simulink model "example_IceStorage"  (R2018b)
settings: Solver=ode45  StartTime=0.0  StopTime=5*24*3600  MaxStep=600  RelTol=1e-4  AbsTol=1e-6  EnableMultiTasking=on
undefined symbols (not defined in the file): path_carnot
libraries: carnot x11
settings Model: Creator=drhf  LastModifiedBy=drhf
settings SolverCC: AutoScaleAbsTol=off  ZeroCrossAlgorithm=Adaptive
settings DataIOCC: LimitDataPoints=on  SaveFormat=Array
settings OptimizationCC: ExpressionDepthLimit=2147483647  LifeSpan=inf
settings DebuggingCC: UnderspecifiedInitializationDetection=Classic  MergeDetectMultiDrivingBlocksExec=none  SolverPrmCheckMsg=warning  StateNameClashWarn=warning  SFUnexpectedBacktrackingDiag=warning  SFNoUnconditionalDefaultTransitionDiag=warning  SFExecutionAtInitializationDiag=none
settings HardwareCC: ProdBitPerPointer=32  ProdBitPerSizeT=32  ProdBitPerPtrDiffT=32  ProdLargestAtomicFloat=None  ProdIntDivRoundTo=Undefined  ProdEndianess=Unspecified  ProdWordSize=32  ProdHWDeviceType=32-bit Generic
settings ModelReferenceCC: PropagateSignalLabelsOutOfModel=off
settings SFSimCC: SimUseLocalCustomCode=off
settings RTWCC: RTWUseLocalCustomCode=off
settings CodeAppCC: StateflowObjectComments=on
settings GRTTargetCC: TargetLangStandard=C89/C90 (ANSI)  GeneratePreprocessorConditionals=Disable all  CombineOutputUpdateFcns=off  GRTInterface=on
settings ConfigComp: CovMetricSettings=dw  CovHtmlReporting=on  CovSaveCumulativeToWorkspaceVar=on  CovSaveSingleToWorkspaceVar=on  CovExternalEMLEnable=off

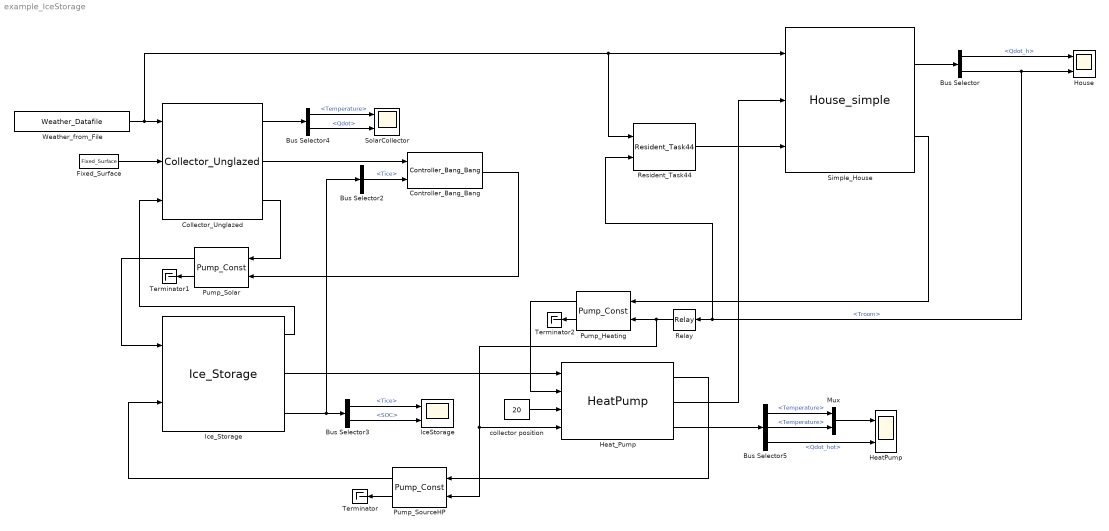
== system example_IceStorage ==
  Bus Selector : BusSelector  OutputSignals=Qdot.Qdot_h,Troom
  Bus Selector2 : BusSelector  OutputSignals=T.Tice
  Bus Selector3 : BusSelector  OutputSignals=T.Tice,SOC
  Bus Selector4 : BusSelector  OutputSignals=THBout.Temperature,Qdot
  Bus Selector5 : BusSelector  OutputSignals=THBin_cold.Temperature,THBout_hot.Temperature,Qdot_hot
  Collector_Unglazed : carnot/Source/Solar_Thermal/Collector_Unglazed  tini=20  Ncollector=1  PathName=fullfile(path_carnot('libsl'), 'Source', 'Solar_Thermal', 'Collector_Unglazed', 'parameter_set')  FileName='DefaultCollectorUnglazed.mat'  userPath=off  userParam=off  acol=2.5  len=2  nodes=10  fta=0.9  eps=0.9  u0l=40  u0c=1  u0g=40  u1l=8  u1c=1  u1g=8  u1e=0.01  hi=200  capa=5000  capf=4000  SensorTimeConstant=10  dplin=5504.4  dpqua=6222.096
      settings: SourceProductName=Carnot
  Controller_Bang_Bang : carnot/Control/Controller_Bang_Bang  deltaTon=5  deltaToff=1  Tmax=95
      settings: SourceProductName=Carnot
  Fixed_Surface : carnot/Weather/Fixed_Surface  colangle=30  colazi=0  colrot=0
      settings: SourceProductName=Carnot
  HeatPump : Scope  NumInputPorts=2
  Heat_Pump : carnot/Source/Heat_Pump/HeatPump  PathName=fullfile(path_carnot('libsl'), 'Source','Heat_Pump','HeatPump','parameter_set')  FileName='DefaultHeatPump.mat'  userPath=off  userParam=off  K=[299.999998982327 -59.9999988176087 12249.9999711932 -6.66666603880034 60.0000010482174 -5.13158332307255e-05 306.666667839537 -115.000000230844 12225.0000010917]  caph=32000  capc=32000  UA=6  relQdotMin=1  linc=10  quac=100  linh=10  quah=100
      settings: SourceProductName=Carnot
  House : Scope  NumInputPorts=2
  IceStorage : Scope  NumInputPorts=2
  Ice_Storage : carnot/Storage/Thermal/Ice_Storage  vol=10  h=2.3  z=3.32-0.12  Lhx_sol=195  Ulen_sol="1500/28/9.5            % 1.5 kW at dT = 9.5 K with a 28 m tube of outer diameter 32 mm"  mpc_sol=1*3500  Lhx_hp=7*50  Ulen_hp="1500/28/9.5            % 1.5 kW at dT = 9.5 K with a 28 m tube of outer diameter 32 mm"  mpc_hp=1*3500  dearth=0.5  cond_ground=2  cp_ground=800  rho_ground=2500  Tmeanoutside=11  deltathetae=9.3  tshift=319  f_ice=0  t_ini=15
      settings: SourceProductName=Carnot
  Mux : Mux  Inputs=2
  Pump_Heating : carnot/Hydraulics/Pump_Const  mdotmax=1200/3600  dia=0.0157  p0=3e5  fluid_id=Water  mix=0  mix2=0  mix3=0  UA=3  mcp=4000  Tini=20  e0=10  e1=10  e2=-1
      settings: SourceProductName=Carnot
  Pump_Solar : carnot/Hydraulics/Pump_Const  mdotmax=1200/3600  dia=0.0157  p0=3e5  fluid_id=Water  mix=0  mix2=0  mix3=0  UA=3  mcp=4000  Tini=20  e0=10  e1=10  e2=-1
      settings: SourceProductName=Carnot
  Pump_SourceHP : carnot/Hydraulics/Pump_Const  mdotmax=2000/3600  dia=0.0157  p0=3e5  fluid_id=Water  mix=0  mix2=0  mix3=0  UA=3  mcp=4000  Tini=20  e0=10  e1=10  e2=-1
      settings: SourceProductName=Carnot
  Relay : Relay  OnSwitchValue=20.2  OffSwitchValue=19.8  OnOutputValue=0  OffOutputValue=1
  Resident_Task44 : carnot/Load/Houses/Resident_Task44  period=24*3600  rep_seq_te=[0 1 6 7 8 9 11 12 13 18 19 20 22 23]*3600  rep_seq_de=[1 5 1 1 1 2 1 1 4 2 1 2 1 1]*3600  rep_seq_ye=[105 55 392.5 457.5 420 55 250 55 120 170 615 420 442.5 355]  rep_seq_to=[0 6 7 8 9 11 12 13 14 15 17 18 20 21 22]*3600  rep_seq_do=[6 1 1 1 2 1 1 1 1 2 1 2 1 1 2]*3600  rep_seq_yo=[4 2 3 2 0 1 3 2 1 0 1 2 4 3 4]*60  Topen=24  Tclose=23  TrAboveTa=2  TaTooCold=12  timeFIR=24  TaIni=12  starttime=8  stoptime=22  TroomShadeOn=23.8  TroomShadeOff=22.8  SolarShadeOn=300  SolarShadeOff=200  max_shade=1  CalcAirComp=off  mdotCO2=0  mdotH2O=0  mdotVOC=0
      settings: SourceProductName=Carnot
  Simple_House : carnot/Load/Houses/House_simple  tini=20  dtroom=inf  Tmeaninside=23.8  deltathetai=3.8  Tmeanoutside=11  deltathetae=9.3  tshift=319*3600  PathName=fullfile(path_carnot('libsl'), 'Load', 'Houses', 'House_simple', 'parameter_set')  FileName='<user defined>'  userPath=off  userParam=on  Ahabit=140  Hroom=2.5  slabwidth=10  slablength=7  dwall=0.4  UAwall=100  capa=500000  utot=0.183  gammat=0  cond_ground=2  cp_ground=800  rho_ground=2500  Awindow=[12 4 3 4]  AziWin=[0 90 -180 -90]  Uwindow=[2 2 2 2]  Gwindow=[0.5 0.5 0.5 0.5]  alpha=10  H=1.2  W=1  Nwin=4  Ventilationrate=0.4  Heatrecovery=0  pnom=10000  dtnom=12.5  expo=0.8  mcap=500*4812  lin=100  qua=100
      settings: SourceProductName=Carnot
  SolarCollector : Scope  NumInputPorts=2
  Terminator : Terminator
  Terminator1 : Terminator
  Terminator2 : Terminator
  Weather_from_File : carnot/Weather/Weather_Datafile  PathName=path_carnot('data')  FileName='DE_TRY2010_04_averageYear.mat'  UserParam=off  VariableName=DE_TRY2010_04_averageYear  SampleTime=3600
      settings: SourceProductName=Carnot
  collector position : Constant  Value=20
  wires:
  Bus Selector/2 -> House/2, Resident_Task44/2, Relay/1  "<Troom>"
  Heat_Pump/2 -> Simple_House/2
  Simple_House/1 -> Bus Selector/1
  Simple_House/2 -> Pump_Heating/1
  Pump_Heating/1 -> Heat_Pump/2
  Relay/1 -> Pump_Heating/2, Pump_SourceHP/2, Heat_Pump/4
  Ice_Storage/2 -> Heat_Pump/1
  Collector_Unglazed/3 -> Pump_Solar/1
  Pump_Solar/1 -> Ice_Storage/1
  Ice_Storage/1 -> Collector_Unglazed/3
  Heat_Pump/1 -> Pump_SourceHP/1
  Ice_Storage/3 -> Bus Selector3/1, Bus Selector2/1
  Controller_Bang_Bang/1 -> Pump_Solar/2
  Collector_Unglazed/2 -> Controller_Bang_Bang/1
  Bus Selector2/1 -> Controller_Bang_Bang/2  "<Tice>"
  Pump_SourceHP/1 -> Ice_Storage/2
  Fixed_Surface/1 -> Collector_Unglazed/2
  collector position/1 -> Heat_Pump/3
  Bus Selector3/1 -> IceStorage/1  "<Tice>"
  Bus Selector3/2 -> IceStorage/2  "<SOC>"
  Bus Selector4/1 -> SolarCollector/1  "<Temperature>"
  Bus Selector4/2 -> SolarCollector/2  "<Qdot>"
  Heat_Pump/3 -> Bus Selector5/1
  Bus Selector5/3 -> HeatPump/2  "<Qdot_hot>"
  Bus Selector5/1 -> Mux/1  "<Temperature>"
  Bus Selector5/2 -> Mux/2  "<Temperature>"
  Mux/1 -> HeatPump/1
  Pump_SourceHP/2 -> Terminator/1
  Pump_Solar/2 -> Terminator1/1
  Pump_Heating/2 -> Terminator2/1
  Bus Selector/1 -> House/1  "<Qdot_h>"
  Collector_Unglazed/1 -> Bus Selector4/1
  Resident_Task44/1 -> Simple_House/3
  Weather_from_File/1 -> Resident_Task44/1, Simple_House/1, Collector_Unglazed/1
